simulink model "ManuAideMoi"  (R2020b)
settings: Solver=VariableStepAuto  StartTime=0.0  StopTime=10.0  RelTol=1e-3
settings Model: Creator=hugom  LastModifiedBy=hugom

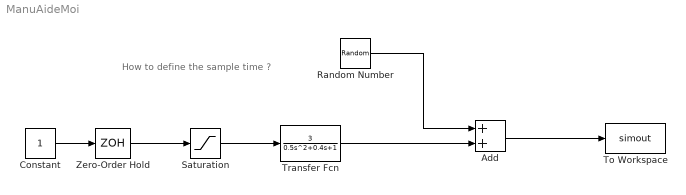
== system ManuAideMoi ==
  note: How to define the sample time ?
  Add : Sum
  Constant : Constant
  Random Number : RandomNumber  Variance=0.15  SampleTime=0.2
  Saturation : Saturate  UpperLimit=0.7  LowerLimit=-0.7
  To Workspace : ToWorkspace  VariableName=simout  SaveFormat=Timeseries  SampleTime=0.2
  Transfer Fcn : TransferFcn  Numerator=[3]  Denominator=[0.5 0.4 1]
  Zero-Order Hold : ZeroOrderHold  SampleTime=0.2
  wires:
  Add/1 -> To Workspace/1
  Transfer Fcn/1 -> Add/2
  Random Number/1 -> Add/1
  Saturation/1 -> Transfer Fcn/1
  Constant/1 -> Zero-Order Hold/1
  Zero-Order Hold/1 -> Saturation/1
